simulink model "twosite_system"  (R2022a)
settings: Solver=ode45  StartTime=-180  StopTime=60*40  RelTol=1e-6
libraries: slpidlib x1
settings Model: Creator=hoshino  LastModifiedBy=hoshino
settings SolverCC: MaxConsecutiveMinStep=10  AlgebraicLoopSolver=TrustRegion
settings DebuggingCC: UnconnectedInputMsg=warning  UnconnectedOutputMsg=warning  UnconnectedLineMsg=warning  SFMachineParentedDataDiag=warning
settings SFSimCC: CustomCodeUndefinedFunction=UseInterfaceOnly
settings RTWCC: DLArmComputeVersion=19.05

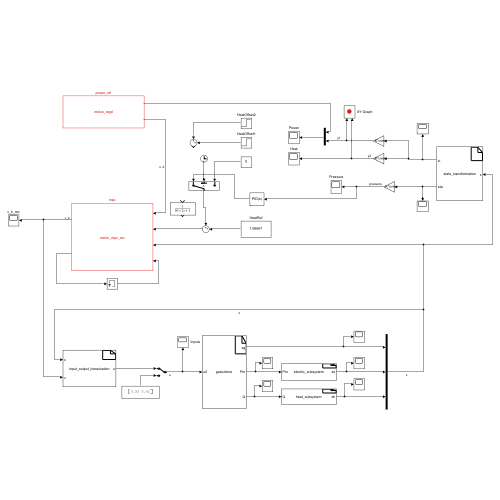
[thumbnail: Simulink's stored preview of the top-level diagram]
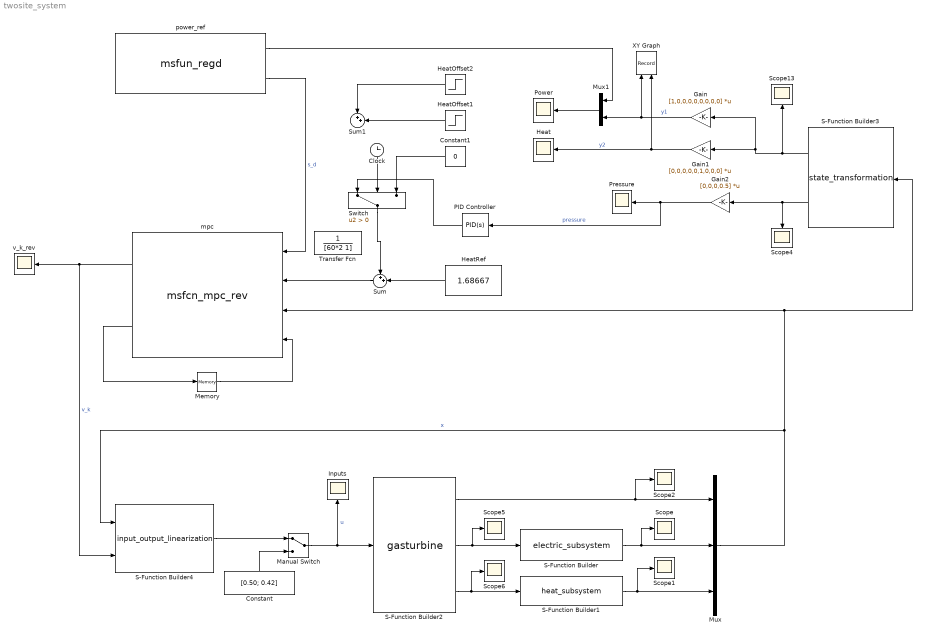
== system twosite_system ==
  Clock : Clock
  Constant : Constant  Value=[0.50; 0.42]
  Constant1 : Constant  Value=0
  Gain : Gain  Gain=[1,0,0,0,0,0,0,0,0]  Multiplication=Matrix(K*u) (u vector)
  Gain1 : Gain  Gain=[0,0,0,0,0,1,0,0,0]  Multiplication=Matrix(K*u) (u vector)
  Gain2 : Gain  Gain=[0,0,0,0.5]  Multiplication=Matrix(K*u) (u vector)
  Heat : Scope
  HeatOffset1 : Step  Time=60*15  Before=0.0  After=-0.0  SampleTime=0
  HeatOffset2 : Step  Time=60*30  After=0.0+0.0  SampleTime=0
  HeatRef : Constant  Value=1.68667
  Inputs : Scope
  Manual Switch : ManualSwitch
  Memory : Memory  InheritSampleTime=on
  Mux : Mux  Inputs=3
  Mux1 : Mux  Inputs=2
  PID Controller : slpidlib/PID Controller  Controller=PID  Form=Parallel  TimeDomain=Continuous-time  UseExternalTs=off  SampleTime=-1  IntegratorMethod=Forward Euler  FilterMethod=Forward Euler  ControllerParametersSource=internal  P=0.01  I=0.001  UseKiTs=off  D=0  N=100  UseFilter=on  TunerSelectOption=Transfer Function Based (PID Tuner App)  InitialConditionSource=internal  InitialConditionForIntegrator=0  InitialConditionForFilter=0  DifferentiatorICPrevScaledInput=0  ExternalReset=none  TrackingMode=off  Kt=1  LimitOutput=off  SatLimitsSource=internal  UpperSaturationLimit=inf  LowerSaturationLimit=-inf  LinearizeAsGain=on  AntiWindupMode=none  Kb=1  POutMin=[]  POutMax=[]  IOutMin=[]  IOutMax=[]  DOutMin=[]  DOutMax=[]  NOutMin=[]  NOutMax=[]  SumOutMin=[]  SumOutMax=[]  SaturationOutMin=[]  SaturationOutMax=[]  PParamMin=[]  PParamMax=[]  IParamMin=[]  IParamMax=[]  DParamMin=[]  DParamMax=[]  NParamMin=[]  NParamMax=[]  KbParamMin=[]  KbParamMax=[]  KtParamMin=[]  KtParamMax=[]  KbOutMin=[]  KbOutMax=[]  KtOutMin=[]  KtOutMax=[]  IntegratorOutMin=[]  IntegratorOutMax=[]  FilterOutMin=[]  FilterOutMax=[]  SumI1OutMin=[]  SumI1OutMax=[]  SumI2OutMin=[]  SumI2OutMax=[]  SumI3OutMin=[]  SumI3OutMax=[]  SumI4OutMin=[]  SumI4OutMax=[]  SumDOutMin=[]  SumDOutMax=[]  DifferentiatorOutMin=[]  DifferentiatorOutMax=[]  FilterDiffOutCoefMin=[]  FilterDiffOutCoefMax=[]  ReciprocalOutMin=[]  ReciprocalOutMax=[]  SumDenOutMin=[]  SumDenOutMax=[]  SumNumOutMin=[]  SumNumOutMax=[]  DivideOutMin=[]  DivideOutMax=[]  UdiffTsProdOutMin=[]  UdiffTsProdOutMax=[]  NTsProdOutMin=[]  NTsProdOutMax=[]  UintegralTsProdOutMin=[]  UintegralTsProdOutMax=[]  UngainTsProdOutMin=[]  UngainTsProdOutMax=[]  IntegratorContinuousStateAttributes=''  IntegratorStateMustResolveToSignalObject=off  IntegratorRTWStateStorageClass=Auto  FilterContinuousStateAttributes=''  FilterStateMustResolveToSignalObject=off  FilterRTWStateStorageClass=Auto  ParallelPVariant=InternalParameters  IdealPVariant=Disabled  IVariant=InternalParameters  DVariant=InternalParameters  IntegratorVariant=Continuous  SatVariant=Disabled  AWVariant=Passthrough  PCopyVariant=Disabled  TRVariant=Disabled  FdbkBlocksVariant=Forward  IdealPFdbkVariant=Disabled  SatFdbkVariant=Disabled  DerivativeFilterVariant=ContFilter  NVariant=InternalParameters  NCopyVariant=Disabled  FilterICVariant=InternalICsFilter  IntegratorICVariant=InternalICs  ExternalResetVariant=Disabled  TRSumVariant=Passthrough  SumFdbkVariant=Disabled  SumVariant=Sum_PID  TsampFilterVariant=InternalTs  TsampNgainVariant=Passthrough  TsampIntegralVariant=Passthrough  ExternalSaturationOutDataTypeStr=Inherit: Same as second input  aMode=0
  Power : Scope
  Pressure : Scope
  S-Function Builder : S-Function  InitFcn=try, set_param(gcb,'FunctionName','electric_subsystem'), end  FunctionName=electric_subsystem  SFunctionModules=electric_subsystem_wrapper cforms  SFunctionDeploymentMode=off  EnableBusSupport=off  mask(S-Function Builder){}
      mask help: Simulink:masks:SFunctionBuilder_MD
      mask init:
      | val = [[.9  0.75 0.75 1 1 .9 .9 1]',[1 1 0.75 0.75 .9 .9 1 .9]'];try , sys = get_param(gcb,'SfunBuilderFcnName');if isempty(sys), sys = get_param(gcb,'FunctionName'); end,catch, sys = get_param(gcb,'FunctionName'); end
      settings: CopyFcn=set_param(gcbh,'LinkStatus','none')  PreSaveFcn=try, set_param(gcb,'FunctionName','electric_subsystem'), end  OpenFcn=sfunctionwizard(gcbh)
      mask Display: plot(val(:,1),val(:,2)),disp(sys), port_label('input',1,'Pm'), port_label('output',1,'xe')
  S-Function Builder1 : S-Function  InitFcn=try, set_param(gcb,'FunctionName','heat_subsystem'), end  FunctionName=heat_subsystem  SFunctionModules=heat_subsystem_wrapper cforms  SFunctionDeploymentMode=off  EnableBusSupport=off  mask(S-Function Builder){}
      mask help: Simulink:masks:SFunctionBuilder_MD
      mask init: same as twosite_system/S-Function Builder
      settings: CopyFcn=set_param(gcbh,'LinkStatus','none')  PreSaveFcn=try, set_param(gcb,'FunctionName','heat_subsystem'), end  OpenFcn=sfunctionwizard(gcbh)
      mask Display: plot(val(:,1),val(:,2)),disp(sys), port_label('input',1,'Q'), port_label('output',1,'xh')
  S-Function Builder2 : S-Function  InitFcn=try, set_param(gcb,'FunctionName','gasturbine'), end  FunctionName=gasturbine  SFunctionModules=gasturbine_wrapper cforms  SFunctionDeploymentMode=off  EnableBusSupport=off  mask(S-Function Builder){}
      mask help: Simulink:masks:SFunctionBuilder_MD
      mask init: same as twosite_system/S-Function Builder
      settings: CopyFcn=set_param(gcbh,'LinkStatus','none')  PreSaveFcn=try, set_param(gcb,'FunctionName','gasturbine'), end  OpenFcn=sfunctionwizard(gcbh)
      mask Display: plot(val(:,1),val(:,2)),disp(sys),port_label('input',1,'u0'),port_label('output',1,'xg'),port_label('output',2,'Pm'),port_label('output',3,'Q')
  S-Function Builder3 : S-Function  InitFcn=try, set_param(gcb,'FunctionName','state_transformation'), end  FunctionName=state_transformation  SFunctionModules=state_transformation_wrapper cforms  SFunctionDeploymentMode=off  EnableBusSupport=off  mask(S-Function Builder){}
      mask help: Simulink:masks:SFunctionBuilder_MD
      mask init: same as twosite_system/S-Function Builder
      settings: CopyFcn=set_param(gcbh,'LinkStatus','none')  PreSaveFcn=try, set_param(gcb,'FunctionName','state_transformation'), end  OpenFcn=sfunctionwizard(gcbh)
      mask Display: plot(val(:,1),val(:,2)),disp(sys),port_label('input',1,'x'),port_label('output',1,'xi'),port_label('output',2,'eta')
  S-Function Builder4 : S-Function  InitFcn=try, set_param(gcb,'FunctionName','input_output_linearization'), end  FunctionName=input_output_linearization  SFunctionModules=input_output_linearization_wrapper cforms  SFunctionDeploymentMode=off  EnableBusSupport=off  mask(S-Function Builder){}
      mask help: Simulink:masks:SFunctionBuilder_MD
      mask init: same as twosite_system/S-Function Builder
      settings: CopyFcn=set_param(gcbh,'LinkStatus','none')  PreSaveFcn=try, set_param(gcb,'FunctionName','input_output_linearization'), end  OpenFcn=sfunctionwizard(gcbh)
      mask Display: plot(val(:,1),val(:,2)),disp(sys),port_label('input',1,'x'),port_label('input',2,'v'),port_label('output',1,'u')
  Scope{,1..2,4..6,13} (7 alike) : Scope
  Sum : Sum  Inputs=++|
  Sum1 : Sum  Inputs=|++
  Switch : Switch  Criteria=u2 > Threshold  SaturateOnIntegerOverflow=off  InputSameDT=off
  Transfer Fcn : TransferFcn  Denominator=[60*2 1]
  XY Graph : Record  FileSettingsInternal="{\"entries\":[{\"content\":{\"excelSettings\":{\"content\":{},\"type\":\"Streamout.ExcelSettings\"}},\"type\":\"Streamout.FileSettingStorage\",\"uuid\":\"7e2d3f37-9943-4f0d-ac7e-a4f3bbad7586\"}],\"packageUris\":[\"http://schema.mathworks.com/mf0/streamout_blocks/R2020a\"],\"version\":\"1.0\"}"  Layout=[1 1]  SignalsInternal="{\"entries\":[{\"content\":{\"signals\":[{\"content\":{\"blockPath\":[\"twosite_system/XY Graph\"],\"channel\":[],\"dimensions\":[1],\"domain\":\"twosite_system/XY Graph\",\"lineColor\":\"#a2142f\",\"plots\":[1],\"port\":1,\"sid\":[],\"signalID\":52867,\"signalName\":\"y1\"},\"type\":\"RecordBlkView.Signal\",\"uuid\":\"43ce5446-7282-4aef-8a2d-fbd5890c7bc5\"},{\"content\":{\"blockPath\":[\"twosite_system/XY Graph\"],\"channel\":[],\"dimensions\":[1],\"domain\":\"twosite_system/XY Graph\",\"lineColor\":\"#139fff\",\"plots\":[1],\"port\":2,\"sid\":[],\"signalID\":52870,\"signalName\":\"y2\"},\"type\":\"RecordBlkView.Signal\",\"uuid\":\"aece1fb8-8165-4249-9dec-86f9523608f4\"}]},\"type\":\"RecordBlkView.InputSignals\",\"uuid\":\"8097ea42-f508-4d80-8f4d-425117022a00\"}],\"packageUris\":[\"http://schema.mathworks.com/mf0/streamout_blocks/R2020a\"],\"version\":\"1.0\"}"  VisualizationBindings="{\"xyplotplugin\":{\"info\":[{\"series\":[{\"bindingParametersList\":[{\"parameter\":\"X-Axis\",\"signalID\":52867,\"signalName\":\"y1\"},{\"parameter\":\"Y-Axis\",\"signalID\":52870,\"signalName\":\"y2\"}],\"seriesID\":20684}],\"subplotID\":1}]}}"  CompatibilityTag=XY
  mpc : M-S-Function  FunctionName=msfcn_mpc_rev  Parameters=Tstep, Nhorizon, Qz, Rv, Plim, u1max, u2max  mask{Tstep=2.0, Nhorizon=5, Qz=blkdiag( 0.1, eye(4), 0.001, eye(3) ), Rv=0.01*eye(2), Plim=[-50, 50], u1max=1.0, u2max=1.0}
      mask prompts: Qz "WeightQ"; Rv "WeightR"
      mask DialogControl ParameterGroupVar Prompt: パラメーター
  power_ref : M-S-Function  FunctionName=msfun_regd  Parameters=Pnominal, ASamplitude  mask{Pnominal=1.0, ASamplitude=0.4}
      mask DialogControl ParameterGroupVar Prompt: パラメーター
  v_k_rev : Scope
  wires:
  S-Function Builder1/1 -> Mux/3, Scope1/1
  S-Function Builder2/2 -> S-Function Builder/1, Scope5/1
  S-Function Builder2/3 -> Scope6/1, S-Function Builder1/1
  S-Function Builder2/1 -> Mux/1, Scope2/1
  S-Function Builder3/2 -> Scope4/1, Gain2/1
  Constant/1 -> Manual Switch/2
  S-Function Builder3/1 -> Scope13/1, Gain1/1, Gain/1
  power_ref/2 -> mpc/1  "s_d"
  S-Function Builder4/1 -> Manual Switch/1
  S-Function Builder/1 -> Scope/1, Mux/2
  Memory/1 -> mpc/4
  Gain/1 -> XY Graph/1, Mux1/2  "y1"
  Gain1/1 -> Heat/1, XY Graph/2  "y2"
  Gain2/1 -> PID Controller/1, Pressure/1  "pressure"
  power_ref/1 -> Mux1/1
  Mux1/1 -> Power/1
  Mux/1 -> S-Function Builder3/1, mpc/3, S-Function Builder4/1  "x"
  mpc/1 -> v_k_rev/1, S-Function Builder4/2  "v_k"
  mpc/2 -> Memory/1
  Manual Switch/1 -> S-Function Builder2/1, Inputs/1  "u"
  Sum/1 -> mpc/2
  HeatRef/1 -> Sum/2
  HeatOffset1/1 -> Sum1/2
  HeatOffset2/1 -> Sum1/1
  Clock/1 -> Switch/2
  Constant1/1 -> Switch/3
  PID Controller/1 -> Switch/1
  Switch/1 -> Sum/1
